simulink model "test_vacc"  (Simulink 7.4)
settings: Solver=ode45  StartTime=0  StopTime=5000  RelTol=1e-3
libraries: xbsIndex_r4 x12, isi_correlator_lib x4, xps_library x2
settings Model: Creator=wjm  LastModifiedBy=wjm
settings OptimizationCC: InitFltsAndDblsToZero=on

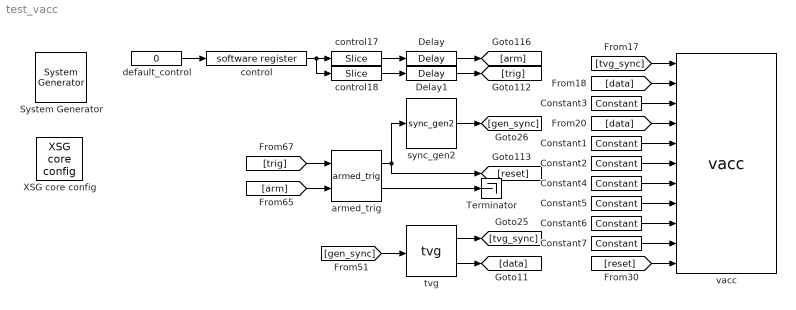
== system test_vacc ==
  " System Generator" : xbsIndex_r4/ System Generator  Tag=genX  SystemSampleTime=-1  xilinxfamily=virtex5  part=xc5vsx95t  speed=-1  package=ff1136  synthesis_tool=XST  clock_wrapper=Clock Enables  directory=./test_vacc/sysgen  testbench=off  simulink_period=1  sysclk_period=5  dcm_input_clock_period=100  incr_netlist=off  trim_vbits=Everywhere in SubSystem  dbl_ovrd=According to Block Masks  core_generation=According to Block Masks  run_coregen=off  deprecated_control=off  eval_field=0  block_type=sysgen
      settings: block_version=10.1.3
  Constant{1..7} (7 alike) : xbsIndex_r4/Constant  arith_type=Signed (2's comp)  const=0  n_bits=32  bin_pt=0  explicit_period=on  period=1  equ=P=C  opselect=C  inp2=PCIN>>17  opr=+  inp1=P  carry=CIN  dbl_ovrd=off  block_type=constant
      settings: block_version=11.4
  Delay : xbsIndex_r4/Delay  en=off  latency=1  dbl_ovrd=off  reg_retiming=on  block_type=delay
      settings: block_version=11.3
  Delay1 : xbsIndex_r4/Delay  en=off  latency=1  dbl_ovrd=off  reg_retiming=on  block_type=delay
      settings: block_version=11.3
  Terminator : Terminator
  XSG core config : xps_library/XSG core config  Tag=xps:xsg  SystemSampleTime=-1  hw_sys=ROACH:sx95t  ibob_linux=off  clk_src=sys_clk2x  iBOB_clk_src=sys_clk  BEE2_ctrl_clk_src=sys_clk  BEE2_usr_clk_src=sys_clk  ROACH_clk_src=sys_clk2x  CORR_clk_src=sys_clk  gpio_clk_io_group=iBOB:sma  gpio_clk_bit_index=0  clk_rate=200  sample_period=1  synthesis_tool=XST  mpc_type=powerpc440_ext
  armed_trig : isi_correlator_lib/armed_trig  SystemSampleTime=-1
  control : xps_library/software register  Tag=xps:sw_reg  SystemSampleTime=-1  io_dir=From Processor  arith_type=Unsigned  bitwidth=32  bin_pt=0  sample_period=1  gw_name=test_vacc_control_user_data_out
  control17 : xbsIndex_r4/Slice  nbits=1  boolean_output=on  mode=Lower Bit Location + Width  bit1=0  base1=MSB of Input  bit0=0  base0=LSB of Input  dbl_ovrd=off  block_type=slice
      settings: infoedit="Extracts a given range of bits from each input sample and presents it at the output.  The output type is ordinarily unsigned with binary point at zero, but can be Boolean when the slice is one bit wide.<P><P>Hardware notes: In hardware this block costs nothing."  block_version=10.1.3
  control18 : xbsIndex_r4/Slice  nbits=1  boolean_output=on  mode=Lower Bit Location + Width  bit1=0  base1=MSB of Input  bit0=1  base0=LSB of Input  dbl_ovrd=off  block_type=slice
      settings: infoedit="Extracts a given range of bits from each input sample and presents it at the output.  The output type is ordinarily unsigned with binary point at zero, but can be Boolean when the slice is one bit wide.<P><P>Hardware notes: In hardware this block costs nothing."  block_version=10.1.3
  default_control : Constant  Value=0  OutDataType=sfix(16)  OutScaling=2^0  SampleTime=1
  sync_gen2 : isi_correlator_lib/sync_gen2  SystemSampleTime=-1
  tvg : isi_correlator_lib/tvg  SystemSampleTime=-1  addr_width=11
  vacc : isi_correlator_lib/vacc  SystemSampleTime=-1  vector_length=8  out_bit_width=27  out_bin_point=4  fanin_latency=3
  wires:
  control18/1 -> Delay1/1
  control17/1 -> Delay/1
  control/1 -> control17/1, control18/1
  Delay1/1 -> [trig]
  default_control/1 -> control/1
  Delay/1 -> [arm]
  armed_trig/1 -> sync_gen2/1, [reset]
  [trig] -> armed_trig/1
  [arm] -> armed_trig/2
  tvg/2 -> [data]
  [gen_sync] -> tvg/1
  tvg/1 -> [tvg_sync]
  sync_gen2/1 -> [gen_sync]
  armed_trig/2 -> Terminator/1
  [tvg_sync] -> vacc/1
  [data] -> vacc/2
  [data] -> vacc/4
  [reset] -> vacc/11
  Constant3/1 -> vacc/3
  Constant1/1 -> vacc/5
  Constant2/1 -> vacc/6
  Constant4/1 -> vacc/7
  Constant5/1 -> vacc/8
  Constant6/1 -> vacc/9
  Constant7/1 -> vacc/10
